simulink model "DJI_Quadcopter_Simulation_2018a"  (R2018a)
settings: Solver=ode45  StartTime=0  StopTime=40  FixedStep=0.02  MaxStep=0.06  RelTol=1e-3  EnableMultiTasking=on
InitFcn:
  | load('batteryModelNew.mat');
  | load('soc_ocv_new.mat');
  | 
  | Q      = battery.QParam; % total capacity in mAh
  | n       = battery.etaParam; % coulombic efficiency
  | M      = battery.MParam; % dynamic hysteresis volts factor
  | Mo     = battery.M0Param; % instant hysteresis volts factor
  | Ro     = battery.R0Param; % internal resistance
  | R       = [battery.RCParam(1)]; % diffusion / warburg impedence, pairs with C
  | C       = [battery.RCParam(2)]; % diffusion / warburg impedence, pairs with R
  | g       = battery.GParam;  % gamma, tunes decay in hysteresis
  | dt      = .01; % delta t
  | eod   = battery.EODParam; % final voltage
  | 
  | if length(R) ~= length(C)
  |     error("R and C must be the same length");
  | end
  | 
  | Arc = zeros(length(R));
  | for i = 1:length(R)
  |     Arc(i,i) = exp(-dt/(R(i)*C(i)));
  | end
  | Brc = zeros(length(R), 1);
  | for i = 1:length(R)
  |     Brc(i,1) = 1 - exp(-dt/(R(i)*C(i)));
  | end
  | k = 1; % timestep
  | Io = .1; % current at time k
  | H(k) = exp(-abs((n(k)*Io(k)*g*dt)/Q));
  | 
  | 
  | %Io = current(1:floor(length(current)/2.5));
  | %Io = current;
  | Io = 0.0;
  | 
  | z = 1.0; % soc
  | Ir = zeros(length(R), 1);
  | h = 0.0;
  | v = ones(length(Io));
  | 
  | 
  | soc = zeros(1, length(Io));
  | v = soc;
model workspace (MAT data in the model file):
  MCOS : class17 (value not decoded)
undefined symbols (not defined in the file): IC, Motor, quadModel, soc_ocv
libraries: simulink x5
(part 2 of 2)

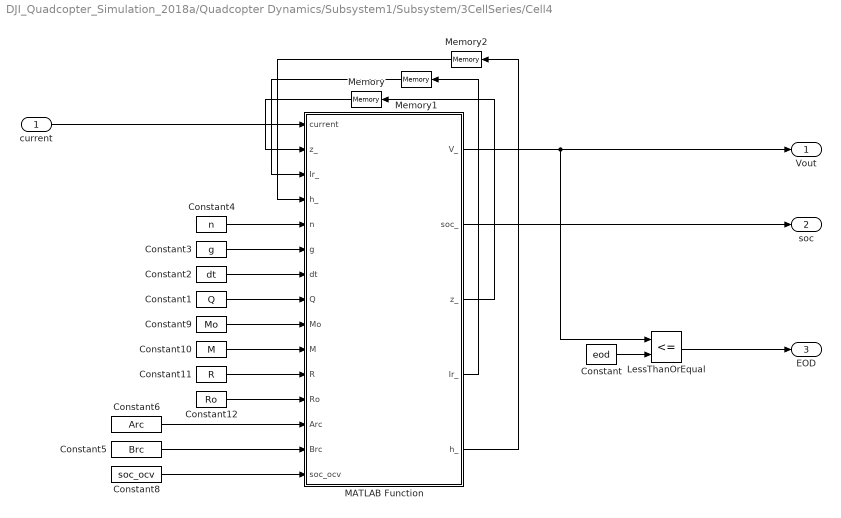
== system DJI_Quadcopter_Simulation_2018a/Quadcopter Dynamics/Subsystem1/Subsystem/3CellSeries/Cell4 ==
  current : Inport
  Constant : Constant  Value=eod
  Constant1 : Constant  Value=Q
  Constant10 : Constant  Value=M
  Constant11 : Constant  Value=R
  Constant12 : Constant  Value=Ro
  Constant2 : Constant  Value=dt
  Constant3 : Constant  Value=g
  Constant4 : Constant  Value=n
  Constant5 : Constant  Value=Brc
  Constant6 : Constant  Value=Arc
  Constant8 : Constant  Value=soc_ocv
  Constant9 : Constant  Value=Mo
  LessThanOrEqual : RelationalOperator  Operator=<=  OutDataTypeStr=boolean  RndMeth=Simplest
  MATLAB Function : MATLAB Function  TreatAsAtomicUnit=on
  Memory : Memory  InitialCondition=1
  Memory1 : Memory
  Memory2 : Memory
  Vout : Outport
  soc : Outport  Port=2
  EOD : Outport  Port=3
  wires:
  MATLAB Function/2(soc_) -> soc/1
  Memory2/1 -> MATLAB Function/4("h_ ")
  Constant11/1 -> MATLAB Function/11(R)
  Constant8/1 -> MATLAB Function/15(soc_ocv)
  Memory/1 -> MATLAB Function/2("z_ ")
  Constant1/1 -> MATLAB Function/8(Q)
  Constant12/1 -> MATLAB Function/12(Ro)
  MATLAB Function/4(Ir_) -> Memory1/1
  Constant5/1 -> MATLAB Function/14(Brc)
  Constant6/1 -> MATLAB Function/13(Arc)
  current/1 -> MATLAB Function/1(current)
  Constant10/1 -> MATLAB Function/10(M)
  Memory1/1 -> MATLAB Function/3("Ir_ ")
  MATLAB Function/3(z_) -> Memory/1
  MATLAB Function/1(V_) -> LessThanOrEqual/1, Vout/1
  MATLAB Function/5(h_) -> Memory2/1
  Constant4/1 -> MATLAB Function/5(n)
  Constant3/1 -> MATLAB Function/6(g)
  Constant9/1 -> MATLAB Function/9(Mo)
  Constant2/1 -> MATLAB Function/7(dt)
  Constant/1 -> LessThanOrEqual/2
  LessThanOrEqual/1 -> EOD/1

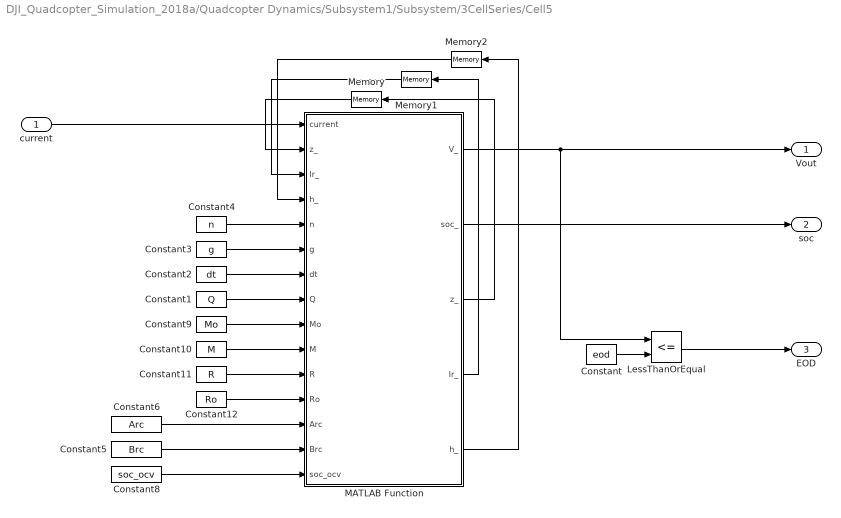
== system DJI_Quadcopter_Simulation_2018a/Quadcopter Dynamics/Subsystem1/Subsystem/3CellSeries/Cell5 ==
  current : Inport
  Constant : Constant  Value=eod
  Constant1 : Constant  Value=Q
  Constant10 : Constant  Value=M
  Constant11 : Constant  Value=R
  Constant12 : Constant  Value=Ro
  Constant2 : Constant  Value=dt
  Constant3 : Constant  Value=g
  Constant4 : Constant  Value=n
  Constant5 : Constant  Value=Brc
  Constant6 : Constant  Value=Arc
  Constant8 : Constant  Value=soc_ocv
  Constant9 : Constant  Value=Mo
  LessThanOrEqual : RelationalOperator  Operator=<=  OutDataTypeStr=boolean  RndMeth=Simplest
  MATLAB Function : MATLAB Function  TreatAsAtomicUnit=on
  Memory : Memory  InitialCondition=1
  Memory1 : Memory
  Memory2 : Memory
  Vout : Outport
  soc : Outport  Port=2
  EOD : Outport  Port=3
  wires:
  MATLAB Function/2(soc_) -> soc/1
  Memory2/1 -> MATLAB Function/4("h_ ")
  Constant11/1 -> MATLAB Function/11(R)
  Constant8/1 -> MATLAB Function/15(soc_ocv)
  Memory/1 -> MATLAB Function/2("z_ ")
  Constant1/1 -> MATLAB Function/8(Q)
  Constant12/1 -> MATLAB Function/12(Ro)
  MATLAB Function/4(Ir_) -> Memory1/1
  Constant5/1 -> MATLAB Function/14(Brc)
  Constant6/1 -> MATLAB Function/13(Arc)
  current/1 -> MATLAB Function/1(current)
  Constant10/1 -> MATLAB Function/10(M)
  Memory1/1 -> MATLAB Function/3("Ir_ ")
  MATLAB Function/3(z_) -> Memory/1
  MATLAB Function/1(V_) -> LessThanOrEqual/1, Vout/1
  MATLAB Function/5(h_) -> Memory2/1
  Constant4/1 -> MATLAB Function/5(n)
  Constant3/1 -> MATLAB Function/6(g)
  Constant9/1 -> MATLAB Function/9(Mo)
  Constant2/1 -> MATLAB Function/7(dt)
  Constant/1 -> LessThanOrEqual/2
  LessThanOrEqual/1 -> EOD/1

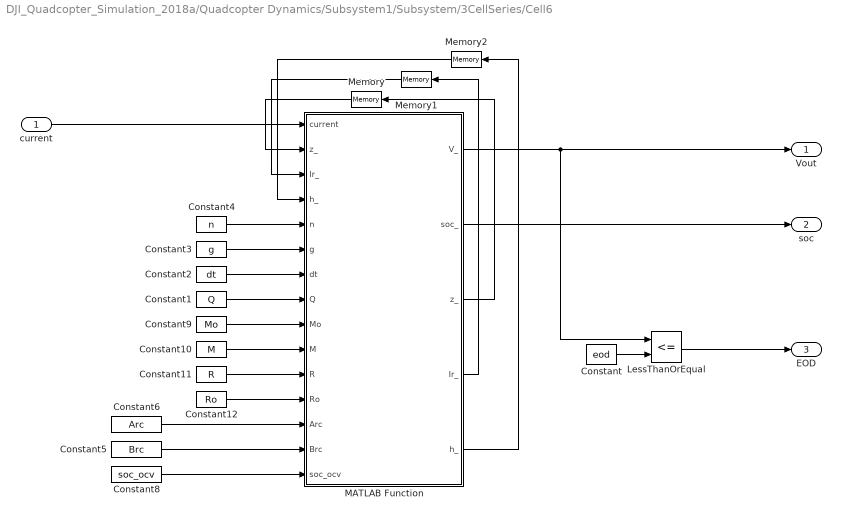
== system DJI_Quadcopter_Simulation_2018a/Quadcopter Dynamics/Subsystem1/Subsystem/3CellSeries/Cell6 ==
  current : Inport
  Constant : Constant  Value=eod
  Constant1 : Constant  Value=Q
  Constant10 : Constant  Value=M
  Constant11 : Constant  Value=R
  Constant12 : Constant  Value=Ro
  Constant2 : Constant  Value=dt
  Constant3 : Constant  Value=g
  Constant4 : Constant  Value=n
  Constant5 : Constant  Value=Brc
  Constant6 : Constant  Value=Arc
  Constant8 : Constant  Value=soc_ocv
  Constant9 : Constant  Value=Mo
  LessThanOrEqual : RelationalOperator  Operator=<=  OutDataTypeStr=boolean  RndMeth=Simplest
  MATLAB Function : MATLAB Function  TreatAsAtomicUnit=on
  Memory : Memory  InitialCondition=1
  Memory1 : Memory
  Memory2 : Memory
  Vout : Outport
  soc : Outport  Port=2
  EOD : Outport  Port=3
  wires:
  MATLAB Function/2(soc_) -> soc/1
  Memory2/1 -> MATLAB Function/4("h_ ")
  Constant11/1 -> MATLAB Function/11(R)
  Constant8/1 -> MATLAB Function/15(soc_ocv)
  Memory/1 -> MATLAB Function/2("z_ ")
  Constant1/1 -> MATLAB Function/8(Q)
  Constant12/1 -> MATLAB Function/12(Ro)
  MATLAB Function/4(Ir_) -> Memory1/1
  Constant5/1 -> MATLAB Function/14(Brc)
  Constant6/1 -> MATLAB Function/13(Arc)
  current/1 -> MATLAB Function/1(current)
  Constant10/1 -> MATLAB Function/10(M)
  Memory1/1 -> MATLAB Function/3("Ir_ ")
  MATLAB Function/3(z_) -> Memory/1
  MATLAB Function/1(V_) -> LessThanOrEqual/1, Vout/1
  MATLAB Function/5(h_) -> Memory2/1
  Constant4/1 -> MATLAB Function/5(n)
  Constant3/1 -> MATLAB Function/6(g)
  Constant9/1 -> MATLAB Function/9(Mo)
  Constant2/1 -> MATLAB Function/7(dt)
  Constant/1 -> LessThanOrEqual/2
  LessThanOrEqual/1 -> EOD/1

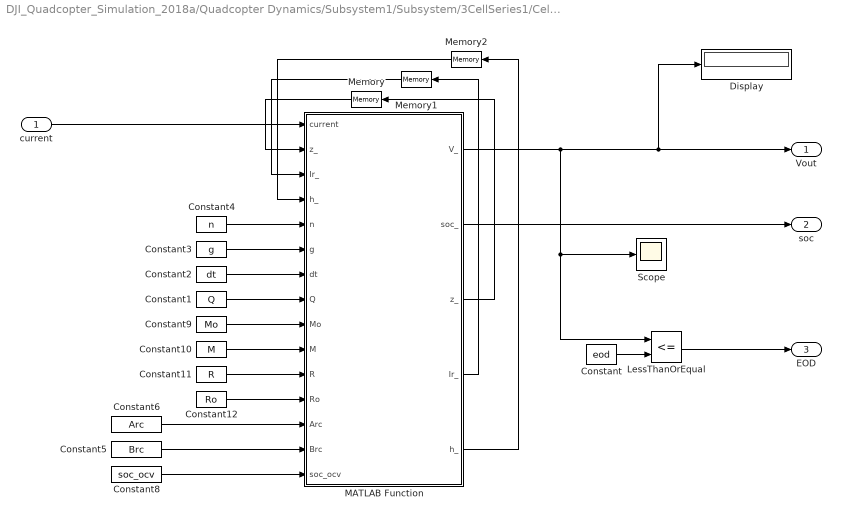
== system DJI_Quadcopter_Simulation_2018a/Quadcopter Dynamics/Subsystem1/Subsystem/3CellSeries1/Cell4 ==
  current : Inport
  Constant : Constant  Value=eod
  Constant1 : Constant  Value=Q
  Constant10 : Constant  Value=M
  Constant11 : Constant  Value=R
  Constant12 : Constant  Value=Ro
  Constant2 : Constant  Value=dt
  Constant3 : Constant  Value=g
  Constant4 : Constant  Value=n
  Constant5 : Constant  Value=Brc
  Constant6 : Constant  Value=Arc
  Constant8 : Constant  Value=soc_ocv
  Constant9 : Constant  Value=Mo
  Display : Display
  LessThanOrEqual : RelationalOperator  Operator=<=  OutDataTypeStr=boolean  RndMeth=Simplest
  MATLAB Function : MATLAB Function  TreatAsAtomicUnit=on
  Memory : Memory  InitialCondition=1
  Memory1 : Memory
  Memory2 : Memory
  Scope : Scope
  Vout : Outport
  soc : Outport  Port=2
  EOD : Outport  Port=3
  wires:
  MATLAB Function/2(soc_) -> soc/1
  Memory2/1 -> MATLAB Function/4("h_ ")
  Constant11/1 -> MATLAB Function/11(R)
  Constant8/1 -> MATLAB Function/15(soc_ocv)
  Memory/1 -> MATLAB Function/2("z_ ")
  Constant1/1 -> MATLAB Function/8(Q)
  Constant12/1 -> MATLAB Function/12(Ro)
  MATLAB Function/4(Ir_) -> Memory1/1
  Constant5/1 -> MATLAB Function/14(Brc)
  Constant6/1 -> MATLAB Function/13(Arc)
  current/1 -> MATLAB Function/1(current)
  Constant10/1 -> MATLAB Function/10(M)
  Memory1/1 -> MATLAB Function/3("Ir_ ")
  MATLAB Function/3(z_) -> Memory/1
  MATLAB Function/1(V_) -> Scope/1, LessThanOrEqual/1, Display/1, Vout/1
  MATLAB Function/5(h_) -> Memory2/1
  Constant4/1 -> MATLAB Function/5(n)
  Constant3/1 -> MATLAB Function/6(g)
  Constant9/1 -> MATLAB Function/9(Mo)
  Constant2/1 -> MATLAB Function/7(dt)
  Constant/1 -> LessThanOrEqual/2
  LessThanOrEqual/1 -> EOD/1

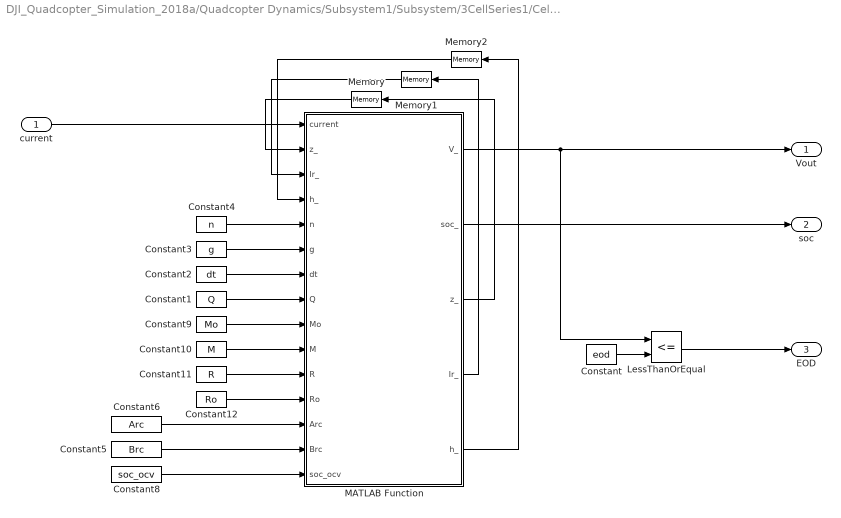
== system DJI_Quadcopter_Simulation_2018a/Quadcopter Dynamics/Subsystem1/Subsystem/3CellSeries1/Cell5 ==
  current : Inport
  Constant : Constant  Value=eod
  Constant1 : Constant  Value=Q
  Constant10 : Constant  Value=M
  Constant11 : Constant  Value=R
  Constant12 : Constant  Value=Ro
  Constant2 : Constant  Value=dt
  Constant3 : Constant  Value=g
  Constant4 : Constant  Value=n
  Constant5 : Constant  Value=Brc
  Constant6 : Constant  Value=Arc
  Constant8 : Constant  Value=soc_ocv
  Constant9 : Constant  Value=Mo
  LessThanOrEqual : RelationalOperator  Operator=<=  OutDataTypeStr=boolean  RndMeth=Simplest
  MATLAB Function : MATLAB Function  TreatAsAtomicUnit=on
  Memory : Memory  InitialCondition=1
  Memory1 : Memory
  Memory2 : Memory
  Vout : Outport
  soc : Outport  Port=2
  EOD : Outport  Port=3
  wires:
  MATLAB Function/2(soc_) -> soc/1
  Memory2/1 -> MATLAB Function/4("h_ ")
  Constant11/1 -> MATLAB Function/11(R)
  Constant8/1 -> MATLAB Function/15(soc_ocv)
  Memory/1 -> MATLAB Function/2("z_ ")
  Constant1/1 -> MATLAB Function/8(Q)
  Constant12/1 -> MATLAB Function/12(Ro)
  MATLAB Function/4(Ir_) -> Memory1/1
  Constant5/1 -> MATLAB Function/14(Brc)
  Constant6/1 -> MATLAB Function/13(Arc)
  current/1 -> MATLAB Function/1(current)
  Constant10/1 -> MATLAB Function/10(M)
  Memory1/1 -> MATLAB Function/3("Ir_ ")
  MATLAB Function/3(z_) -> Memory/1
  MATLAB Function/1(V_) -> LessThanOrEqual/1, Vout/1
  MATLAB Function/5(h_) -> Memory2/1
  Constant4/1 -> MATLAB Function/5(n)
  Constant3/1 -> MATLAB Function/6(g)
  Constant9/1 -> MATLAB Function/9(Mo)
  Constant2/1 -> MATLAB Function/7(dt)
  Constant/1 -> LessThanOrEqual/2
  LessThanOrEqual/1 -> EOD/1

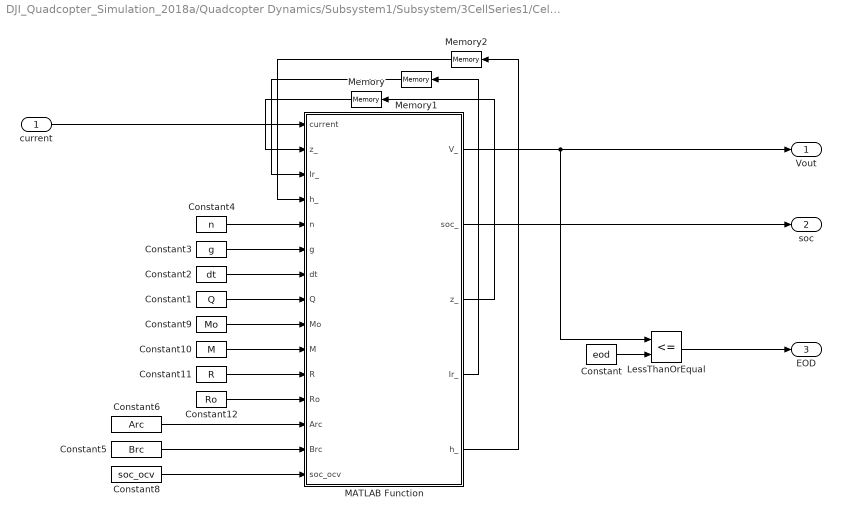
== system DJI_Quadcopter_Simulation_2018a/Quadcopter Dynamics/Subsystem1/Subsystem/3CellSeries1/Cell6 ==
  current : Inport
  Constant : Constant  Value=eod
  Constant1 : Constant  Value=Q
  Constant10 : Constant  Value=M
  Constant11 : Constant  Value=R
  Constant12 : Constant  Value=Ro
  Constant2 : Constant  Value=dt
  Constant3 : Constant  Value=g
  Constant4 : Constant  Value=n
  Constant5 : Constant  Value=Brc
  Constant6 : Constant  Value=Arc
  Constant8 : Constant  Value=soc_ocv
  Constant9 : Constant  Value=Mo
  LessThanOrEqual : RelationalOperator  Operator=<=  OutDataTypeStr=boolean  RndMeth=Simplest
  MATLAB Function : MATLAB Function  TreatAsAtomicUnit=on
  Memory : Memory  InitialCondition=1
  Memory1 : Memory
  Memory2 : Memory
  Vout : Outport
  soc : Outport  Port=2
  EOD : Outport  Port=3
  wires:
  MATLAB Function/2(soc_) -> soc/1
  Memory2/1 -> MATLAB Function/4("h_ ")
  Constant11/1 -> MATLAB Function/11(R)
  Constant8/1 -> MATLAB Function/15(soc_ocv)
  Memory/1 -> MATLAB Function/2("z_ ")
  Constant1/1 -> MATLAB Function/8(Q)
  Constant12/1 -> MATLAB Function/12(Ro)
  MATLAB Function/4(Ir_) -> Memory1/1
  Constant5/1 -> MATLAB Function/14(Brc)
  Constant6/1 -> MATLAB Function/13(Arc)
  current/1 -> MATLAB Function/1(current)
  Constant10/1 -> MATLAB Function/10(M)
  Memory1/1 -> MATLAB Function/3("Ir_ ")
  MATLAB Function/3(z_) -> Memory/1
  MATLAB Function/1(V_) -> LessThanOrEqual/1, Vout/1
  MATLAB Function/5(h_) -> Memory2/1
  Constant4/1 -> MATLAB Function/5(n)
  Constant3/1 -> MATLAB Function/6(g)
  Constant9/1 -> MATLAB Function/9(Mo)
  Constant2/1 -> MATLAB Function/7(dt)
  Constant/1 -> LessThanOrEqual/2
  LessThanOrEqual/1 -> EOD/1

== matlab function DJI_Quadcopter_Simulation_2018a/Quadcopter Dynamics/Motor Dynamics/Subsystem1/motorRotor4/Mechanical part/Propeller model  ==
  data: torque output; rpm input; thrust output
function [torque,thrust] = fcn(rpm)
% angular_velocity in rpm

%coefficient of thrust, empirically derived
coef_t = 2*(10^-15)*rpm^3 - 4*(10^-11)*rpm^2 + 3*(10^-7)*rpm + .1013;
%thrust = coef_t * density of air * velocity^2 * propeller diameter (m) ^4
thrust = coef_t*1.225*(rpm/60)^2*.2^4;
% empirically derived
torque = 4*(10^-14)*rpm^3 +  8*(10^-12)*rpm^2 + 3*(10^-6)*rpm;
end

== matlab function DJI_Quadcopter_Simulation_2018a/Quadcopter Dynamics/Motor Dynamics/Subsystem2/motorRotor4/Mechanical part/Propeller model  ==
  data: torque output; rpm input; thrust output
function [torque,thrust] = fcn(rpm)
% angular_velocity in rpm

%coefficient of thrust, empirically derived
coef_t = 2*(10^-15)*rpm^3 - 4*(10^-11)*rpm^2 + 3*(10^-7)*rpm + .1013;
%thrust = coef_t * density of air * velocity^2 * propeller diameter (m) ^4
thrust = coef_t*1.225*(rpm/60)^2*.2^4;
% empirically derived
torque = 4*(10^-14)*rpm^3 +  8*(10^-12)*rpm^2 + 3*(10^-6)*rpm;
end

== matlab function DJI_Quadcopter_Simulation_2018a/Quadcopter Dynamics/Motor Dynamics/Subsystem3/motorRotor4/Mechanical part/Propeller model  ==
  data: torque output; rpm input; thrust output
function [torque,thrust] = fcn(rpm)
% angular_velocity in rpm

%coefficient of thrust, empirically derived
coef_t = 2*(10^-15)*rpm^3 - 4*(10^-11)*rpm^2 + 3*(10^-7)*rpm + .1013;
%thrust = coef_t * density of air * velocity^2 * propeller diameter (m) ^4
thrust = coef_t*1.225*(rpm/60)^2*.2^4;
% empirically derived
torque = 4*(10^-14)*rpm^3 +  8*(10^-12)*rpm^2 + 3*(10^-6)*rpm;
end

== matlab function DJI_Quadcopter_Simulation_2018a/Quadcopter Dynamics/Subsystem1/Subsystem/3CellSeries/Cell4/MATLAB Function ==
  data: current input; V_ output; z_ input; Ir_ input; h_ input; soc_ output; z_ output; Ir_ output; h_ output; n input; g input; dt input; Q input; Mo input; M input; R input; Ro input; Arc input; Brc input; soc_ocv input
function [V_, soc_, z_, Ir_, h_]= batterySim(current, z_, Ir_, h_, n, g, dt, Q, Mo, M, R, Ro, Arc, Brc, soc_ocv)
    soc_ = 1.0;
    V_ = 4.2;
    z_dot = z_ - ((n*dt)/Q)*current;
    Ir_dot = Arc*Ir_ + Brc*current;
    H = exp(-abs((n*current*g*dt)/Q));
    h_dot = H*h_ + (H-1)*sign(current);
    z_ = z_dot;
    Ir_ = Ir_dot;
    h_ = h_dot;
    soc_ = (z_ + 31.8816) /(1.0 + 31.8816);
    idx = ceil(soc_*100) +1;
    V_ = (soc_ocv(idx) + Mo*sign(current) + M*h_ - sum(R*Ir_) - Ro*current);

== matlab function DJI_Quadcopter_Simulation_2018a/Quadcopter Dynamics/Subsystem1/Subsystem/3CellSeries/Cell5/MATLAB Function ==
  data: current input; V_ output; z_ input; Ir_ input; h_ input; soc_ output; z_ output; Ir_ output; h_ output; n input; g input; dt input; Q input; Mo input; M input; R input; Ro input; Arc input; Brc input; soc_ocv input
function [V_, soc_, z_, Ir_, h_]= batterySim(current, z_, Ir_, h_, n, g, dt, Q, Mo, M, R, Ro, Arc, Brc, soc_ocv)
    soc_ = 1.0;
    V_ = 4.2;
    z_dot = z_ - ((n*dt)/Q)*current;
    Ir_dot = Arc*Ir_ + Brc*current;
    H = exp(-abs((n*current*g*dt)/Q));
    h_dot = H*h_ + (H-1)*sign(current);
    z_ = z_dot;
    Ir_ = Ir_dot;
    h_ = h_dot;
    soc_ = (z_ + 31.8816) /(1.0 + 31.8816);
    idx = ceil(soc_*100) +1;
    V_ = (soc_ocv(idx) + Mo*sign(current) + M*h_ - sum(R*Ir_) - Ro*current);

== matlab function DJI_Quadcopter_Simulation_2018a/Quadcopter Dynamics/Subsystem1/Subsystem/3CellSeries/Cell6/MATLAB Function ==
  data: current input; V_ output; z_ input; Ir_ input; h_ input; soc_ output; z_ output; Ir_ output; h_ output; n input; g input; dt input; Q input; Mo input; M input; R input; Ro input; Arc input; Brc input; soc_ocv input
function [V_, soc_, z_, Ir_, h_]= batterySim(current, z_, Ir_, h_, n, g, dt, Q, Mo, M, R, Ro, Arc, Brc, soc_ocv)
    soc_ = 1.0;
    V_ = 4.2;
    z_dot = z_ - ((n*dt)/Q)*current;
    Ir_dot = Arc*Ir_ + Brc*current;
    H = exp(-abs((n*current*g*dt)/Q));
    h_dot = H*h_ + (H-1)*sign(current);
    z_ = z_dot;
    Ir_ = Ir_dot;
    h_ = h_dot;
    soc_ = (z_ + 31.8816) /(1.0 + 31.8816);
    idx = ceil(soc_*100) +1;
    V_ = (soc_ocv(idx) + Mo*sign(current) + M*h_ - sum(R*Ir_) - Ro*current);

== matlab function DJI_Quadcopter_Simulation_2018a/Quadcopter Dynamics/Subsystem1/Subsystem/3CellSeries1/Cell4/MATLAB Function ==
  data: current input; V_ output; z_ input; Ir_ input; h_ input; soc_ output; z_ output; Ir_ output; h_ output; n input; g input; dt input; Q input; Mo input; M input; R input; Ro input; Arc input; Brc input; soc_ocv input
function [V_, soc_, z_, Ir_, h_]= batterySim(current, z_, Ir_, h_, n, g, dt, Q, Mo, M, R, Ro, Arc, Brc, soc_ocv)
    soc_ = 1.0;
    V_ = 4.2;
    z_dot = z_ - ((n*dt)/Q)*current;
    Ir_dot = Arc*Ir_ + Brc*current;
    H = exp(-abs((n*current*g*dt)/Q));
    h_dot = H*h_ + (H-1)*sign(current);
    z_ = z_dot;
    Ir_ = Ir_dot;
    h_ = h_dot;
    soc_ = (z_ + 31.8816) /(1.0 + 31.8816);
    idx = ceil(soc_*100) +1;
    V_ = (soc_ocv(idx) + Mo*sign(current) + M*h_ - sum(R*Ir_) - Ro*current);

== matlab function DJI_Quadcopter_Simulation_2018a/Quadcopter Dynamics/Subsystem1/Subsystem/3CellSeries1/Cell5/MATLAB Function ==
  data: current input; V_ output; z_ input; Ir_ input; h_ input; soc_ output; z_ output; Ir_ output; h_ output; n input; g input; dt input; Q input; Mo input; M input; R input; Ro input; Arc input; Brc input; soc_ocv input
function [V_, soc_, z_, Ir_, h_]= batterySim(current, z_, Ir_, h_, n, g, dt, Q, Mo, M, R, Ro, Arc, Brc, soc_ocv)
    soc_ = 1.0;
    V_ = 4.2;
    z_dot = z_ - ((n*dt)/Q)*current;
    Ir_dot = Arc*Ir_ + Brc*current;
    H = exp(-abs((n*current*g*dt)/Q));
    h_dot = H*h_ + (H-1)*sign(current);
    z_ = z_dot;
    Ir_ = Ir_dot;
    h_ = h_dot;
    soc_ = (z_ + 31.8816) /(1.0 + 31.8816);
    idx = ceil(soc_*100) +1;
    V_ = (soc_ocv(idx) + Mo*sign(current) + M*h_ - sum(R*Ir_) - Ro*current);

== matlab function DJI_Quadcopter_Simulation_2018a/Quadcopter Dynamics/Subsystem1/Subsystem/3CellSeries1/Cell6/MATLAB Function ==
  data: current input; V_ output; z_ input; Ir_ input; h_ input; soc_ output; z_ output; Ir_ output; h_ output; n input; g input; dt input; Q input; Mo input; M input; R input; Ro input; Arc input; Brc input; soc_ocv input
function [V_, soc_, z_, Ir_, h_]= batterySim(current, z_, Ir_, h_, n, g, dt, Q, Mo, M, R, Ro, Arc, Brc, soc_ocv)
    soc_ = 1.0;
    V_ = 4.2;
    z_dot = z_ - ((n*dt)/Q)*current;
    Ir_dot = Arc*Ir_ + Brc*current;
    H = exp(-abs((n*current*g*dt)/Q));
    h_dot = H*h_ + (H-1)*sign(current);
    z_ = z_dot;
    Ir_ = Ir_dot;
    h_ = h_dot;
    soc_ = (z_ + 31.8816) /(1.0 + 31.8816);
    idx = ceil(soc_*100) +1;
    V_ = (soc_ocv(idx) + Mo*sign(current) + M*h_ - sum(R*Ir_) - Ro*current);

== matlab function DJI_Quadcopter_Simulation_2018a/Quadcopter Dynamics/Subsystem1/Subsystem/MATLAB Function ==
  data: u input; a output; b output
function [a,b]= fcn(u)

a = u/2;
b = u/2;

== matlab function DJI_Quadcopter_Simulation_2018a/Quadcopter Dynamics/Motor Dynamics/Subsystem/motorRotor4/Mechanical part/Propeller model  ==
  data: torque output; rpm input; thrust output
function [torque,thrust] = fcn(rpm)
% angular_velocity in rpm

%coefficient of thrust, empirically derived
coef_t = 2*(10^-15)*rpm^3 - 4*(10^-11)*rpm^2 + 3*(10^-7)*rpm + .1013;
%thrust = coef_t * density of air * velocity^2 * propeller diameter (m) ^4
thrust = coef_t*1.225*(rpm/60)^2*.2^4;
% empirically derived
torque = 4*(10^-14)*rpm^3 +  8*(10^-12)*rpm^2 + 3*(10^-6)*rpm;
end
